simulink model "testmodel2017b"  (R2017b)
settings: Solver=FixedStepDiscrete  StartTime=0.0  StopTime=1000  FixedStep=srate  RelTol=1e-3
PreLoadFcn:
  | model_startup;
model workspace (MAT data in the model file):
  CD_IFBK_GAIN = Simulink.Parameter
  CD_IFBK_GAIN.Value = 0.00279947916667
  CD_IFBK_GAIN.DataType = 'single'
  CD_IFBK_GAIN.Dimensions = [1 1]
  CD_INTEGRATOR_RESET_I = Simulink.Parameter
  CD_INTEGRATOR_RESET_I.Value = 0.01
  CD_INTEGRATOR_RESET_I.DataType = 'single'
  CD_INTEGRATOR_RESET_I.Dimensions = [1 1]
  CD_PRECISION_REF_NOM = Simulink.Parameter
  CD_PRECISION_REF_NOM.Value = 511
  CD_PRECISION_REF_NOM.DataType = 'single'
  CD_PRECISION_REF_NOM.Dimensions = [1 1]
  CD_SOLENOID_RES = Simulink.Parameter
  CD_SOLENOID_RES.Value = 6.1803
  CD_SOLENOID_RES.DataType = 'single'
  CD_SOLENOID_RES.Dimensions = [1 1]
  CD_VBATTERY_GAIN = Simulink.Parameter
  CD_VBATTERY_GAIN.Value = 0.0293360157816
  CD_VBATTERY_GAIN.DataType = 'single'
  CD_VBATTERY_GAIN.Dimensions = [1 1]
  CD_VBATTERY_NOM = Simulink.Parameter
  CD_VBATTERY_NOM.Value = 13.5
  CD_VBATTERY_NOM.DataType = 'single'
  CD_VBATTERY_NOM.Dimensions = [1 1]
  OnPower = Simulink.Signal
  OnPower.DataType = 'boolean'
  OnPower.Dimensions = -1
  OnPower.DimensionsMode = 'auto'
  OnPower.Complexity = 'auto'
  OnPower.SampleTime = -1
  OnPower.SamplingMode = 'auto'
  numOutputs = 6
  srate = 0.001
values from neighbouring files (symbols this model uses):
  CMD_INVERTER_GOTO_OPERATIONAL = Bobcat.Parameter; CreateDefine( CMD_INVERTER_GOTO_OPERATIONAL ,uint8(1) ,'Define' ,'defines.h' )    [enums.m]
  CMD_INVERTER_GOTO_READY = Bobcat.Parameter; CreateDefine( CMD_INVERTER_GOTO_READY       ,uint8(2) ,'Define' ,'defines.h' )    [enums.m]
  CMD_INVERTER_GOTO_STOP = Bobcat.Parameter; CreateDefine( CMD_INVERTER_GOTO_STOP        ,uint8(0) ,'Define' ,'defines.h' )    [enums.m]
  CMD_INVERTER_RUN_FWD = Bobcat.Parameter; CreateDefine( CMD_INVERTER_RUN_FWD          ,uint8(3) ,'Define' ,'defines.h' )    [enums.m]
  INVERTER_CONNECTED = Bobcat.Parameter; CreateDefine( INVERTER_CONNECTED   ,uint8(1) ,'Define' ,'defines.h' )    [enums.m]
  INVERTER_OPERATIONAL = Bobcat.Parameter; CreateDefine( INVERTER_OPERATIONAL ,uint8(2) ,'Define' ,'defines.h' )    [enums.m]
  INVERTER_READY = Bobcat.Parameter; CreateDefine( INVERTER_READY       ,uint8(3) ,'Define' ,'defines.h' )    [enums.m]
  INVERTER_RUN_FWD = Bobcat.Parameter; CreateDefine( INVERTER_RUN_FWD     ,uint8(4) ,'Define' ,'defines.h' )    [enums.m]
  INVERTER_STOP = Bobcat.Parameter; CreateDefine( INVERTER_STOP        ,uint8(0) ,'Define' ,'defines.h' )    [enums.m]
undefined symbols (not defined in the file or in its folder): a, b, c, sigbuilder_block
libraries: simulink x9, hdlsllib x1
CloseFcn:
  | model_end;
settings Model: NumberOfSteps=20000  Creator=cswenson  LastModifiedBy=mmaffeo
settings DataIOCC: SaveOutput=off  SaveTime=off  ReturnWorkspaceOutputs=on
settings OptimizationCC: DefaultParameterBehavior=Inlined  InlineInvariantSignals=on  EnhancedBackFolding=on  PassReuseOutputArgsAs=Individual arguments  StateBitsets=on  DataBitsets=on  LifeSpan=inf  OptimizeBlockOrder=speed  DifferentSizesBufferReuse=on
settings DebuggingCC: ReadBeforeWriteMsg=DisableAll  WriteAfterWriteMsg=DisableAll  WriteAfterReadMsg=DisableAll  AlgebraicLoopMsg=error  ArtificialAlgebraicLoopMsg=error  SaveWithParameterizedLinksMsg=error  BlockPriorityViolationMsg=error  SolverPrmCheckMsg=error  InheritedTsInSrcMsg=error  MultiTaskDSMMsg=none  SigSpecEnsureSampleTimeMsg=error  IntegerOverflowMsg=error  ParameterUnderflowMsg=warning  ParameterTunabilityLossMsg=error  UnderSpecifiedDataTypeMsg=error  UnnecessaryDatatypeConvMsg=warning  VectorMatrixConversionMsg=error  FcnCallInpInsideContextMsg=warning  UnconnectedInputMsg=error  UnconnectedOutputMsg=error  UnconnectedLineMsg=error  SFcnCompatibilityMsg=error  BusObjectLabelMismatch=error  RootOutportRequireBusObject=error  AssertControl=DisableAll  ModelReferenceIOMsg=error  ModelReferenceIOMismatchMessage=error  UnknownTsInhSupMsg=error  ModelReferenceDataLoggingMessage=error  StateNameClashWarn=warning  SFUnexpectedBacktrackingDiag=warning  SFNoUnconditionalDefaultTransitionDiag=warning  SFExecutionAtInitializationDiag=none
settings HardwareCC: ProdBitPerPointer=32  ProdBitPerSizeT=32  ProdBitPerPtrDiffT=32  ProdLargestAtomicInteger=Long  ProdLargestAtomicFloat=Double  ProdWordSize=32  ProdHWDeviceType=ARM Compatible->ARM Cortex  TargetBitPerPointer=64  TargetBitPerSizeT=64  TargetBitPerPtrDiffT=64  TargetLongLongMode=on  TargetIntDivRoundTo=Zero  TargetEndianess=LittleEndian  TargetWordSize=64  TargetHWDeviceType=MATLAB Host
settings ModelReferenceCC: UpdateModelReferenceTargets=IfOutOfDate  PropagateSignalLabelsOutOfModel=off
settings SFSimCC: SimUserSources=SendMsgNow_Blank.cpp  SimUserIncludeDirs=functions  SFSimEcho=off  MATLABDynamicMemAlloc=off
settings SFSimCC: SimCustomHeaderCode=|
  | #include "SendMsgNow.h"
  | #define uint8_t unsigned char
settings RTWCC: SystemTargetFile=bobcat_ert.tlc  GenCodeOnly=on  GenerateMakefile=off  TemplateMakefile=ert_default_tmf  Description=Bobcat Embedded Target derived from RTW-EC  GenerateReport=on  RTWVerbose=off  IncludeHyperlinkInReport=on  LaunchReport=on  PortableWordSizes=on  TargetLang=C++  GenerateTraceInfo=on  GenerateTraceReport=on  GenerateTraceReportSl=on  GenerateTraceReportSf=on  GenerateTraceReportEml=on  GenerateCodeMetricsReport=on  GenerateCodeReplacementReport=on
settings RTWCC: CustomHeaderCode=|
  | #include "cdata.h"
  | #include "ap_can.h"
  | #include "SendMsgNow.h"
  | #include "ap_eeprom.h"
  | #include "ap_bservice_CAN04.h"
settings CodeAppCC: ForceParamTrailComments=on  IgnoreCustomStorageClasses=off  IgnoreTestpoints=on  MangleLength=4  StateflowObjectComments=on  InternalIdentifier=Classic  ReqsInCode=on
settings STFCustomTargetCC: MultiwordLength=256  IncludeMdlTerminateFcn=off  CombineOutputUpdateFcns=on  ERTCustomFileBanners=on  SupportNonFinite=off  SupportComplex=off  SupportNonInlinedSFcns=off  MATLABClassNameForMDSCustomization=Simulink.SoftwareTarget.ERTCustomization  GRTInterface=off  SystemTargetFile=bobcat_ert.tlc
settings ERTTargetCC: ParMdlRefBuildCompliant=off  CompOptLevelCompliant=off  ConcurrentExecutionCompliant=off  IncludeMdlTerminateFcn=off  SupportNonFinite=off  SupportComplex=off  SupportContinuousTime=on  RemoveResetFunc=off  ModelStepFunctionPrototypeControlCompliant=off  CPPClassGenCompliant=off  UseToolchainInfoCompliant=off  InlinedParameterPlacement=NonHierarchical  ERTSrcFileBannerTemplate=bobcat_ert_template.cgt  ERTHdrFileBannerTemplate=bobcat_ert_template.cgt  ERTDataSrcFileTemplate=bobcat_ert_template.cgt  ERTDataHdrFileTemplate=bobcat_ert_template.cgt  ERTCustomFileTemplate=bobcat_file_process.tlc  PreserveExpressionOrder=on  PreserveIfCondition=on  ConvertIfToSwitch=off  SuppressUnreachableDefaultCases=off
settings ConfigComp: CovScope=ReferencedModels  CovIncludeTopModel=off  CovMetricSettings=dw  CovHtmlReporting=on  CovSaveCumulativeToWorkspaceVar=on  CovSaveSingleToWorkspaceVar=on  CovExternalEMLEnable=off  CovSFcnEnable=off

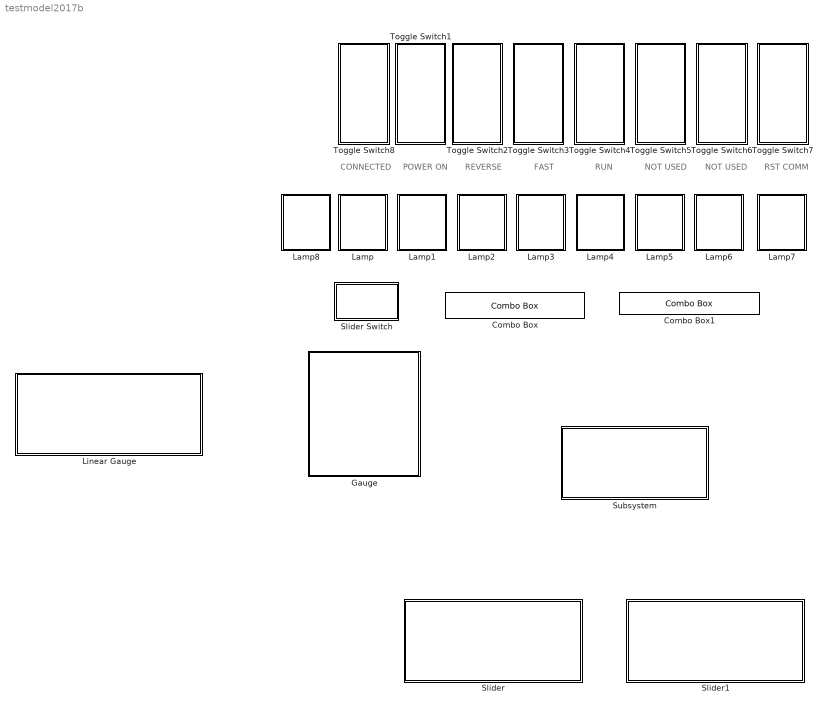
== system testmodel2017b ==
  note: CONNECTED
  note: POWER ON
  note: REVERSE
  note: FAST
  note: RST COMM
  note: RUN
  note: NOT USED
  note: NOT USED
  Combo Box : ComboBox  WebBlockId=8705  ModelName=testmodel2017b  LabelPosition=Top  ShowInitialText=on  SelectedLabel=stop
      settings: Values={{'stop', 'connected', 'operational', 'ready', 'run fwd', 'run rev'}, [0 1 2 3 4 5]}
  Combo Box1 : ComboBox  WebBlockId=8718  ModelName=testmodel2017b  LabelPosition=Hide  ShowInitialText=on  SelectedLabel=Go stop
      settings: Values={{'Go stop', 'Go connected', 'Go operational', 'Go ready', 'Run fwd', 'Run rev'}, [0 1 2 3 4 5]}
  Gauge : Subsystem  DialogController=hmiCreateDDGDialog  IsWebBlock=on  mask(MWDashboardBlock){webBlockId=ca701e44-4673-470a-9dd6-e67335b96dcc, webBlockType=circulargauge, ShowInLibBrowser=on, ShowInitialText=on, HMISrcModelName=testmodel2017b}
      mask prompts: webBlockId "WebBlock Id"; webBlockType "WebBlock Type"; HMISrcModelName "Source Model"
      mask help: SimulinkHMI:dialogs:CircularGaugeDialogDesc
      mask Help: helpview([docroot '/mapfiles/simulink.map'], 'hmi_gauge')
      mask Display:
      | if strcmp(get_param(bdroot(gcb),'BlockDiagramType'), 'library')
      |     image([(matlabroot) '/toolbox/simulink/hmi/icons/CircularGauge.png']);
      | end
  Lamp : Subsystem  DialogController=hmiCreateDDGDialog  IsWebBlock=on  mask(MWDashboardBlock){webBlockId=3d03b230-6085-4f28-82bc-8c8f72340ffd, webBlockType=lamp, ShowInLibBrowser=on, ShowInitialText=on, HMISrcModelName=testmodel2017b}
      mask prompts: webBlockId "WebBlock Id"; webBlockType "WebBlock Type"; HMISrcModelName "Source Model"
      mask help: Display a color that reflects an input value.
      mask Help: helpview([docroot '/mapfiles/simulink.map'], 'hmi_lamp')
      mask Display:
      | if strcmp(get_param(bdroot(gcb),'BlockDiagramType'),'library')
      |  image([(matlabroot) '/toolbox/simulink/hmi/icons/Lamp.png'])
      | end
  Lamp1 : Subsystem  DialogController=hmiCreateDDGDialog  IsWebBlock=on  mask(MWDashboardBlock){webBlockId=3b8bfb2c-1eac-4315-b443-895d23544263, webBlockType=lamp, ShowInLibBrowser=on, ShowInitialText=on, HMISrcModelName=testmodel2017b}
      mask prompts: webBlockId "WebBlock Id"; webBlockType "WebBlock Type"; HMISrcModelName "Source Model"
      mask help: Display a color that reflects an input value.
      mask Help: helpview([docroot '/mapfiles/simulink.map'], 'hmi_lamp')
      mask Display:
      | if strcmp(get_param(bdroot(gcb),'BlockDiagramType'),'library')
      |  image([(matlabroot) '/toolbox/simulink/hmi/icons/Lamp.png'])
      | end
  Lamp2 : Subsystem  DialogController=hmiCreateDDGDialog  IsWebBlock=on  mask(MWDashboardBlock){webBlockId=1077b2a3-7ee6-4687-bbb4-987db73cae4f, webBlockType=lamp, ShowInLibBrowser=on, ShowInitialText=on, HMISrcModelName=testmodel2017b}
      mask prompts: webBlockId "WebBlock Id"; webBlockType "WebBlock Type"; HMISrcModelName "Source Model"
      mask help: Display a color that reflects an input value.
      mask Help: helpview([docroot '/mapfiles/simulink.map'], 'hmi_lamp')
      mask Display:
      | if strcmp(get_param(bdroot(gcb),'BlockDiagramType'),'library')
      |  image([(matlabroot) '/toolbox/simulink/hmi/icons/Lamp.png'])
      | end
  Lamp3 : Subsystem  DialogController=hmiCreateDDGDialog  IsWebBlock=on  mask(MWDashboardBlock){webBlockId=5a2165d5-e830-43a3-9a69-8f3d244f6c12, webBlockType=lamp, ShowInLibBrowser=on, ShowInitialText=on, HMISrcModelName=testmodel2017b}
      mask prompts: webBlockId "WebBlock Id"; webBlockType "WebBlock Type"; HMISrcModelName "Source Model"
      mask help: Display a color that reflects an input value.
      mask Help: helpview([docroot '/mapfiles/simulink.map'], 'hmi_lamp')
      mask Display:
      | if strcmp(get_param(bdroot(gcb),'BlockDiagramType'),'library')
      |  image([(matlabroot) '/toolbox/simulink/hmi/icons/Lamp.png'])
      | end
  Lamp4 : Subsystem  DialogController=hmiCreateDDGDialog  IsWebBlock=on  mask(MWDashboardBlock){webBlockId=2857e801-db19-4a7d-a036-5bbc043663b6, webBlockType=lamp, ShowInLibBrowser=on, ShowInitialText=on, HMISrcModelName=testmodel2017b}
      mask prompts: webBlockId "WebBlock Id"; webBlockType "WebBlock Type"; HMISrcModelName "Source Model"
      mask help: Display a color that reflects an input value.
      mask Help: helpview([docroot '/mapfiles/simulink.map'], 'hmi_lamp')
      mask Display:
      | if strcmp(get_param(bdroot(gcb),'BlockDiagramType'),'library')
      |  image([(matlabroot) '/toolbox/simulink/hmi/icons/Lamp.png'])
      | end
  Lamp5 : Subsystem  DialogController=hmiCreateDDGDialog  IsWebBlock=on  mask(MWDashboardBlock){webBlockId=4482e485-1c61-4683-8091-409276114980, webBlockType=lamp, ShowInLibBrowser=on, ShowInitialText=on, HMISrcModelName=testmodel2017b}
      mask prompts: webBlockId "WebBlock Id"; webBlockType "WebBlock Type"; HMISrcModelName "Source Model"
      mask help: Display a color that reflects an input value.
      mask Help: helpview([docroot '/mapfiles/simulink.map'], 'hmi_lamp')
      mask Display:
      | if strcmp(get_param(bdroot(gcb),'BlockDiagramType'),'library')
      |  image([(matlabroot) '/toolbox/simulink/hmi/icons/Lamp.png'])
      | end
  Lamp6 : Subsystem  DialogController=hmiCreateDDGDialog  IsWebBlock=on  mask(MWDashboardBlock){webBlockId=9855c58a-8830-4368-a696-a0d1540bb0ee, webBlockType=lamp, ShowInLibBrowser=on, ShowInitialText=on, HMISrcModelName=testmodel2017b}
      mask prompts: webBlockId "WebBlock Id"; webBlockType "WebBlock Type"; HMISrcModelName "Source Model"
      mask help: Display a color that reflects an input value.
      mask Help: helpview([docroot '/mapfiles/simulink.map'], 'hmi_lamp')
      mask Display:
      | if strcmp(get_param(bdroot(gcb),'BlockDiagramType'),'library')
      |  image([(matlabroot) '/toolbox/simulink/hmi/icons/Lamp.png'])
      | end
  Lamp7 : Subsystem  DialogController=hmiCreateDDGDialog  IsWebBlock=on  mask(MWDashboardBlock){webBlockId=786d7a47-f623-41eb-b7ff-b095192b59d1, webBlockType=lamp, ShowInLibBrowser=on, ShowInitialText=on, HMISrcModelName=testmodel2017b}
      mask prompts: webBlockId "WebBlock Id"; webBlockType "WebBlock Type"; HMISrcModelName "Source Model"
      mask help: Display a color that reflects an input value.
      mask Help: helpview([docroot '/mapfiles/simulink.map'], 'hmi_lamp')
      mask Display:
      | if strcmp(get_param(bdroot(gcb),'BlockDiagramType'),'library')
      |  image([(matlabroot) '/toolbox/simulink/hmi/icons/Lamp.png'])
      | end
  Lamp8 : Subsystem  DialogController=hmiCreateDDGDialog  IsWebBlock=on  mask(MWDashboardBlock){webBlockId=bc0dacb4-7449-4962-80f3-d142238d4a2f, webBlockType=lamp, ShowInLibBrowser=on, ShowInitialText=on, HMISrcModelName=testmodel2017b}
      mask prompts: webBlockId "WebBlock Id"; webBlockType "WebBlock Type"; HMISrcModelName "Source Model"
      mask help: Display a color that reflects an input value.
      mask Help: helpview([docroot '/mapfiles/simulink.map'], 'hmi_lamp')
      mask Display:
      | if strcmp(get_param(bdroot(gcb),'BlockDiagramType'),'library')
      |  image([(matlabroot) '/toolbox/simulink/hmi/icons/Lamp.png'])
      | end
  Linear Gauge : Subsystem  DialogController=hmiCreateDDGDialog  IsWebBlock=on  mask(MWDashboardBlock){webBlockId=7f63c228-2e19-4776-af30-abd338e55317, webBlockType=lineargauge, ShowInLibBrowser=on, ShowInitialText=on, HMISrcModelName=testmodel2017b}
      mask prompts: webBlockId "WebBlock Id"; webBlockType "WebBlock Type"; HMISrcModelName "Source Model"
      mask help: SimulinkHMI:dialogs:LinearGaugeDialogDesc
      mask Help: helpview([docroot '/mapfiles/simulink.map'], 'hmi_linear_gauge')
      mask Display:
      | if strcmp(get_param(bdroot(gcb),'BlockDiagramType'), 'library')
      |     image([(matlabroot) '/toolbox/simulink/hmi/icons/LinearGauge.png']);
      | end
  Slider : Subsystem  DialogController=hmiCreateDDGDialog  IsWebBlock=on  mask(MWDashboardBlock){webBlockId=fa958995-471b-4ba4-bec5-340cf4a0c4a4, webBlockType=slider, ShowInLibBrowser=on, ShowInitialText=on, HMISrcModelName=testmodel2017b}
      mask prompts: webBlockId "WebBlock Id"; webBlockType "WebBlock Type"; HMISrcModelName "Source Model"
      mask help: SimulinkHMI:dialogs:SliderDialogDesc
      mask Help: helpview([docroot '/mapfiles/simulink.map'], 'hmi_slider')
      mask Display:
      | if strcmp(get_param(bdroot(gcb),'BlockDiagramType'), 'library')
      |     image([(matlabroot) '/toolbox/simulink/hmi/icons/Slider.png']);
      | end
  Slider Switch : Subsystem  DialogController=hmiCreateDDGDialog  IsWebBlock=on  mask(MWDashboardBlock){webBlockId=e8f953b1-b3fd-4705-a0b6-97bfe8724c95, webBlockType=sliderswitch, ShowInLibBrowser=on, ShowInitialText=on, HMISrcModelName=testmodel2017b}
      mask prompts: webBlockId "WebBlock Id"; webBlockType "WebBlock Type"; HMISrcModelName "Source Model"
      mask help: Set on/off value to tune parameters or variables.
      mask Help: helpview([docroot '/mapfiles/simulink.map'], 'hmi_switch')
      mask Display:
      | if strcmp(get_param(bdroot(gcb),'BlockDiagramType'),'library')
      |  image([(matlabroot) '/toolbox/simulink/hmi/icons/SliderSwitch.png'])
      | end
  Slider1 : Subsystem  DialogController=hmiCreateDDGDialog  IsWebBlock=on  mask(MWDashboardBlock){webBlockId=517096a1-4060-40ba-819b-9a3d476b2f75, webBlockType=slider, ShowInLibBrowser=on, ShowInitialText=on, HMISrcModelName=testmodel2017b}
      mask prompts: webBlockId "WebBlock Id"; webBlockType "WebBlock Type"; HMISrcModelName "Source Model"
      mask help: SimulinkHMI:dialogs:SliderDialogDesc
      mask Help: helpview([docroot '/mapfiles/simulink.map'], 'hmi_slider')
      mask Display:
      | if strcmp(get_param(bdroot(gcb),'BlockDiagramType'), 'library')
      |     image([(matlabroot) '/toolbox/simulink/hmi/icons/Slider.png']);
      | end
  Subsystem : Subsystem
  Toggle Switch1 : Subsystem  DialogController=hmiCreateDDGDialog  IsWebBlock=on  mask(MWDashboardBlock){webBlockId=47589691-0491-44e5-b52c-3802481a810c, webBlockType=toggleswitch, ShowInLibBrowser=on, ShowInitialText=on, HMISrcModelName=testmodel2017b}
      mask prompts: webBlockId "WebBlock Id"; webBlockType "WebBlock Type"; HMISrcModelName "Source Model"
      mask help: SimulinkHMI:dialogs:SwitchDialogDesc
      mask Help: helpview([docroot '/mapfiles/simulink.map'], 'hmi_toggle_switch')
      mask Display:
      | if strcmp(get_param(bdroot(gcb),'BlockDiagramType'), 'library')
      |     image([(matlabroot) '/toolbox/simulink/hmi/icons/ToggleSwitch.png']);
      | end
  Toggle Switch2 : Subsystem  DialogController=hmiCreateDDGDialog  IsWebBlock=on  mask(MWDashboardBlock){webBlockId=03349644-d7f0-4194-b582-00e40be6aa1b, webBlockType=toggleswitch, ShowInLibBrowser=on, ShowInitialText=on, HMISrcModelName=testmodel2017b}
      mask prompts: webBlockId "WebBlock Id"; webBlockType "WebBlock Type"; HMISrcModelName "Source Model"
      mask help: SimulinkHMI:dialogs:SwitchDialogDesc
      mask Help: helpview([docroot '/mapfiles/simulink.map'], 'hmi_toggle_switch')
      mask Display:
      | if strcmp(get_param(bdroot(gcb),'BlockDiagramType'), 'library')
      |     image([(matlabroot) '/toolbox/simulink/hmi/icons/ToggleSwitch.png']);
      | end
  Toggle Switch3 : Subsystem  DialogController=hmiCreateDDGDialog  IsWebBlock=on  mask(MWDashboardBlock){webBlockId=8be4c630-fc00-43e9-b3e7-282d6444acbb, webBlockType=toggleswitch, ShowInLibBrowser=on, ShowInitialText=on, HMISrcModelName=testmodel2017b}
      mask prompts: webBlockId "WebBlock Id"; webBlockType "WebBlock Type"; HMISrcModelName "Source Model"
      mask help: SimulinkHMI:dialogs:SwitchDialogDesc
      mask Help: helpview([docroot '/mapfiles/simulink.map'], 'hmi_toggle_switch')
      mask Display:
      | if strcmp(get_param(bdroot(gcb),'BlockDiagramType'), 'library')
      |     image([(matlabroot) '/toolbox/simulink/hmi/icons/ToggleSwitch.png']);
      | end
  Toggle Switch4 : Subsystem  DialogController=hmiCreateDDGDialog  IsWebBlock=on  mask(MWDashboardBlock){webBlockId=669c9247-3514-4664-88b6-ae32ca600e88, webBlockType=toggleswitch, ShowInLibBrowser=on, ShowInitialText=on, HMISrcModelName=testmodel2017b}
      mask prompts: webBlockId "WebBlock Id"; webBlockType "WebBlock Type"; HMISrcModelName "Source Model"
      mask help: SimulinkHMI:dialogs:SwitchDialogDesc
      mask Help: helpview([docroot '/mapfiles/simulink.map'], 'hmi_toggle_switch')
      mask Display:
      | if strcmp(get_param(bdroot(gcb),'BlockDiagramType'), 'library')
      |     image([(matlabroot) '/toolbox/simulink/hmi/icons/ToggleSwitch.png']);
      | end
  Toggle Switch5 : Subsystem  DialogController=hmiCreateDDGDialog  IsWebBlock=on  mask(MWDashboardBlock){webBlockId=9df9911a-db6a-4f88-9175-2bee3af0034b, webBlockType=toggleswitch, ShowInLibBrowser=on, ShowInitialText=on, HMISrcModelName=testmodel2017b}
      mask prompts: webBlockId "WebBlock Id"; webBlockType "WebBlock Type"; HMISrcModelName "Source Model"
      mask help: SimulinkHMI:dialogs:SwitchDialogDesc
      mask Help: helpview([docroot '/mapfiles/simulink.map'], 'hmi_toggle_switch')
      mask Display:
      | if strcmp(get_param(bdroot(gcb),'BlockDiagramType'), 'library')
      |     image([(matlabroot) '/toolbox/simulink/hmi/icons/ToggleSwitch.png']);
      | end
  Toggle Switch6 : Subsystem  DialogController=hmiCreateDDGDialog  IsWebBlock=on  mask(MWDashboardBlock){webBlockId=26248c20-b423-42ea-b6b6-d3060b4fe5f6, webBlockType=toggleswitch, ShowInLibBrowser=on, ShowInitialText=on, HMISrcModelName=testmodel2017b}
      mask prompts: webBlockId "WebBlock Id"; webBlockType "WebBlock Type"; HMISrcModelName "Source Model"
      mask help: SimulinkHMI:dialogs:SwitchDialogDesc
      mask Help: helpview([docroot '/mapfiles/simulink.map'], 'hmi_toggle_switch')
      mask Display:
      | if strcmp(get_param(bdroot(gcb),'BlockDiagramType'), 'library')
      |     image([(matlabroot) '/toolbox/simulink/hmi/icons/ToggleSwitch.png']);
      | end
  Toggle Switch7 : Subsystem  DialogController=hmiCreateDDGDialog  IsWebBlock=on  mask(MWDashboardBlock){webBlockId=519b3b3b-eed3-4fa3-8c24-ef273513dd86, webBlockType=toggleswitch, ShowInLibBrowser=on, ShowInitialText=on, HMISrcModelName=testmodel2017b}
      mask prompts: webBlockId "WebBlock Id"; webBlockType "WebBlock Type"; HMISrcModelName "Source Model"
      mask help: SimulinkHMI:dialogs:SwitchDialogDesc
      mask Help: helpview([docroot '/mapfiles/simulink.map'], 'hmi_toggle_switch')
      mask Display:
      | if strcmp(get_param(bdroot(gcb),'BlockDiagramType'), 'library')
      |     image([(matlabroot) '/toolbox/simulink/hmi/icons/ToggleSwitch.png']);
      | end
  Toggle Switch8 : Subsystem  DialogController=hmiCreateDDGDialog  IsWebBlock=on  mask(MWDashboardBlock){webBlockId=17c79f1b-60e0-4136-926c-46730ae39f4c, webBlockType=toggleswitch, ShowInLibBrowser=on, ShowInitialText=on, HMISrcModelName=testmodel2017b}
      mask prompts: webBlockId "WebBlock Id"; webBlockType "WebBlock Type"; HMISrcModelName "Source Model"
      mask help: SimulinkHMI:dialogs:SwitchDialogDesc
      mask Help: helpview([docroot '/mapfiles/simulink.map'], 'hmi_toggle_switch')
      mask Display:
      | if strcmp(get_param(bdroot(gcb),'BlockDiagramType'), 'library')
      |     image([(matlabroot) '/toolbox/simulink/hmi/icons/ToggleSwitch.png']);
      | end

== system testmodel2017b/Gauge ==

== system testmodel2017b/Lamp ==

== system testmodel2017b/Lamp1 ==

== system testmodel2017b/Lamp2 ==

== system testmodel2017b/Lamp3 ==

== system testmodel2017b/Lamp4 ==

== system testmodel2017b/Lamp5 ==

== system testmodel2017b/Lamp6 ==

== system testmodel2017b/Lamp7 ==

== system testmodel2017b/Lamp8 ==

== system testmodel2017b/Linear Gauge ==

== system testmodel2017b/Slider ==

== system testmodel2017b/Slider Switch ==

== system testmodel2017b/Slider1 ==

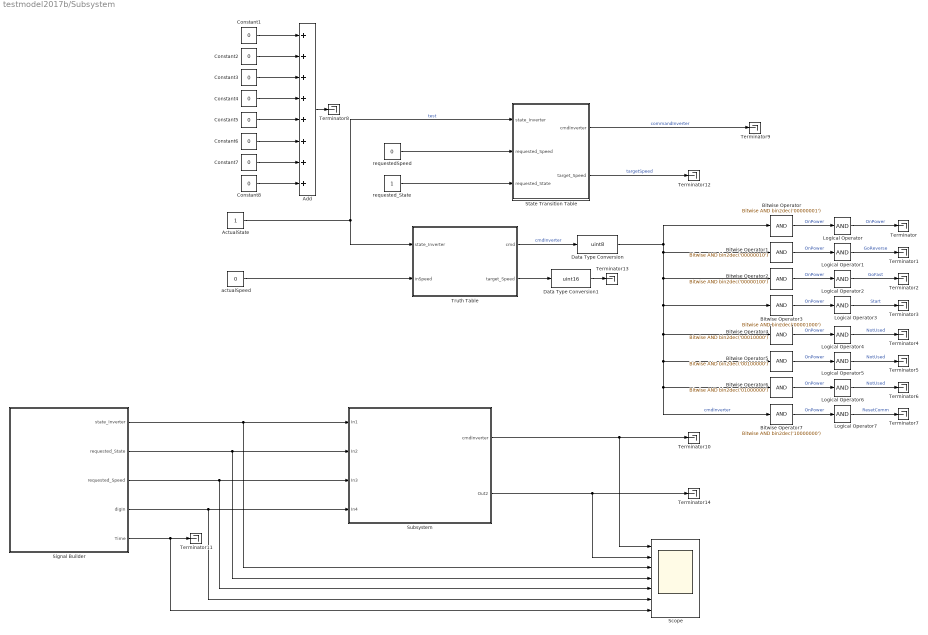
== system testmodel2017b/Subsystem ==
  ActualState : Constant  OutDataTypeStr=uint8
  Add : Sum  Inputs=++++++++  OutDataTypeStr=uint8
  Bitwise Operator : simulink/Logic and Bit Operations/Bitwise Operator  logicop=AND  UseBitMask=on  BitMask=bin2dec('00000001')  BitMaskRealWorld=Stored Integer
  Bitwise Operator1 : simulink/Logic and Bit Operations/Bitwise Operator  logicop=AND  UseBitMask=on  BitMask=bin2dec('00000010')  BitMaskRealWorld=Stored Integer
  Bitwise Operator2 : simulink/Logic and Bit Operations/Bitwise Operator  logicop=AND  UseBitMask=on  BitMask=bin2dec('00000100')  BitMaskRealWorld=Stored Integer
  Bitwise Operator3 : simulink/Logic and Bit Operations/Bitwise Operator  logicop=AND  UseBitMask=on  BitMask=bin2dec('00001000')  BitMaskRealWorld=Stored Integer
  Bitwise Operator4 : simulink/Logic and Bit Operations/Bitwise Operator  logicop=AND  UseBitMask=on  BitMask=bin2dec('00010000')  BitMaskRealWorld=Stored Integer
  Bitwise Operator5 : simulink/Logic and Bit Operations/Bitwise Operator  logicop=AND  UseBitMask=on  BitMask=bin2dec('00100000')  BitMaskRealWorld=Stored Integer
  Bitwise Operator6 : simulink/Logic and Bit Operations/Bitwise Operator  logicop=AND  UseBitMask=on  BitMask=bin2dec('01000000')  BitMaskRealWorld=Stored Integer
  Bitwise Operator7 : simulink/Logic and Bit Operations/Bitwise Operator  logicop=AND  UseBitMask=on  BitMask=bin2dec('10000000')  BitMaskRealWorld=Stored Integer
  Constant{1..8} (8 alike) : Constant  Value=0
  Data Type Conversion : DataTypeConversion  OutDataTypeStr=uint8
  Data Type Conversion1 : DataTypeConversion  OutDataTypeStr=uint16
  Logical Operator{,1..7} (8 alike) : Logic  Inputs=1  AllPortsSameDT=off  OutDataTypeStr=boolean
  Scope : Scope  NumInputPorts=7
  Signal Builder : Subsystem  Tag=STV Subsys  LoadFcn=sigbuilder_block('load',[-1536 0 1536 808.8 ]);  StartFcn=sigbuilder_block('start');  StopFcn=sigbuilder_block('stop');  ClipboardFcn=sigbuilder_block('clipboard');  mask(Sigbuilder block){tuvar=[0:10]}
      mask help: Simulink:masks:SigbuilderBlock_MD
      mask init:
      | if ~strcmp(get_param(bdroot(gcbh),'SimulationStatus'),'stopped') tuvar = sigbuilder_block('maskInit'); end
      settings: CopyFcn=sigbuilder_block('copy');  DeleteFcn=sigbuilder_block('delete');  ModelCloseFcn=sigbuilder_block('modelClose');  PreSaveFcn=sigbuilder_block('preSave');  PauseFcn=sigbuilder_block('pause');  ContinueFcn=sigbuilder_block('continue');  NameChangeFcn=sigbuilder_block('namechange');  OpenFcn=sigbuilder_block('open',[437.6 199.2 550.4 400 ]);  CloseFcn=sigbuilder_block('close');
      mask Display: plot(0, 0, 100, 100,[2, 2, 32, 32, 2], [68, 8, 8, 68, 68],[32, 2], [38, 38], [32, 19, 2],[53, 60, 44], [32, 17, 17, 2],[16, 16, 31, 31]);txt = getActiveGroup(gcbh);text(2, 100, txt,'verticalAlignment', 'top');
  State Transition Table : State Transition Table  TreatAsAtomicUnit=on
  Subsystem : Subsystem
  Terminator{,1..14} (15 alike) : Terminator
  Truth Table : Truth Table  TreatAsAtomicUnit=on
  actualSpeed : Constant  Value=0  OutDataTypeStr=uint16
  requestedSpeed : Constant  Value=0  OutDataTypeStr=uint16
  requested_State : Constant  OutDataTypeStr=uint8
  wires:
  ActualState/1 -> Truth Table/1(state_Inverter), State Transition Table/1(state_Inverter)  "test"
  Constant1/1 -> Add/1
  Constant7/1 -> Add/7
  Constant5/1 -> Add/5
  Constant6/1 -> Add/6
  Constant8/1 -> Add/8
  Constant4/1 -> Add/4
  Constant2/1 -> Add/2
  Constant3/1 -> Add/3
  Logical Operator/1 -> Terminator/1  "OnPower"
  Logical Operator1/1 -> Terminator1/1  "GoReverse"
  Logical Operator4/1 -> Terminator4/1  "NotUsed"
  Logical Operator5/1 -> Terminator5/1  "NotUsed"
  Logical Operator6/1 -> Terminator6/1  "NotUsed"
  Logical Operator7/1 -> Terminator7/1  "ResetComm"
  Data Type Conversion/1 -> Bitwise Operator7/1, Bitwise Operator6/1, Bitwise Operator5/1, Bitwise Operator4/1, Bitwise Operator3/1, Bitwise Operator2/1, Bitwise Operator1/1, Bitwise Operator/1  "cmdInverter"
  Bitwise Operator/1 -> Logical Operator/1  "OnPower"
  Bitwise Operator1/1 -> Logical Operator1/1  "OnPower"
  Bitwise Operator2/1 -> Logical Operator2/1  "OnPower"
  Bitwise Operator3/1 -> Logical Operator3/1  "OnPower"
  Logical Operator2/1 -> Terminator2/1  "GoFast"
  Logical Operator3/1 -> Terminator3/1  "Start"
  Bitwise Operator7/1 -> Logical Operator7/1  "OnPower"
  Bitwise Operator4/1 -> Logical Operator4/1  "OnPower"
  Bitwise Operator6/1 -> Logical Operator6/1  "OnPower"
  Bitwise Operator5/1 -> Logical Operator5/1  "OnPower"
  Add/1 -> Terminator8/1
  actualSpeed/1 -> Truth Table/2(inSpeed)
  Truth Table/1(cmd) -> Data Type Conversion/1  "cmdInverter"
  Truth Table/2(target_Speed) -> Data Type Conversion1/1
  requested_State/1 -> State Transition Table/3(requested_State)
  State Transition Table/1(cmdInverter) -> Terminator9/1  "commandInverter"
  requestedSpeed/1 -> State Transition Table/2(requested_Speed)
  Signal Builder/2(requested_State) -> Subsystem/2(In2), Scope/4
  Signal Builder/3(requested_Speed) -> Subsystem/3(In3), Scope/5
  Signal Builder/1(state_Inverter) -> Subsystem/1(In1), Scope/3
  Signal Builder/5(Time) -> Scope/7, Terminator11/1
  State Transition Table/2(target_Speed) -> Terminator12/1  "targetSpeed"
  Data Type Conversion1/1 -> Terminator13/1
  Signal Builder/4(digIn) -> Subsystem/4(In4), Scope/6
  Subsystem/2(Out2) -> Terminator14/1, Scope/2
  Subsystem/1(cmdInverter) -> Terminator10/1, Scope/1

== system testmodel2017b/Toggle Switch1 ==

== system testmodel2017b/Toggle Switch2 ==

== system testmodel2017b/Toggle Switch3 ==

== system testmodel2017b/Toggle Switch4 ==

== system testmodel2017b/Toggle Switch5 ==

== system testmodel2017b/Toggle Switch6 ==

== system testmodel2017b/Toggle Switch7 ==

== system testmodel2017b/Toggle Switch8 ==

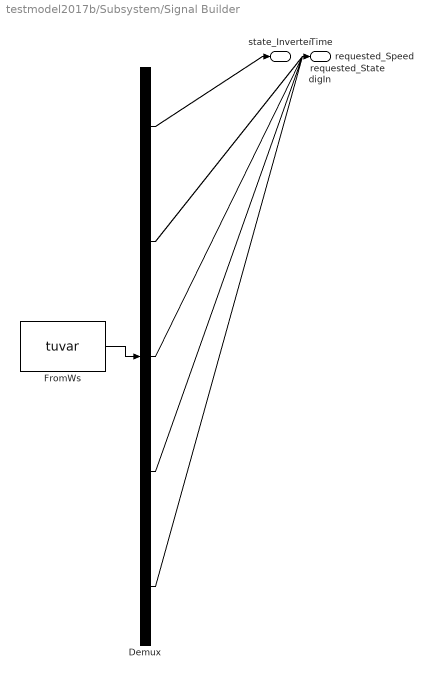
== system testmodel2017b/Subsystem/Signal Builder ==
  Demux : Demux  Tag=STV Demux  Outputs=5
  FromWs : FromWorkspace  Tag=STV FromWs  VariableName=tuvar  SampleTime=0
      SigBuilderData=|
      | common.afterFinalStr = 'Extrapolate'
      | common.sampleTime = 0
      | dataSet(1).timeRange = [0 1000]
      | dataSet(1).name = 'Normal Sequence'
      | dataSet(2).timeRange = [0 1000]
      | dataSet(2).name = 'EmergenzyStop'
      | dataSet(3).timeRange = [0 1000]
      | dataSet(3).name = 'SeatBar'
      | sbobj.Name = 'Signal Builder'
      | sbobj.Groups(1).Name = 'Normal Sequence'
      | sbobj.Groups(1).Signals(1).Name = 'state_Inverter'
      | sbobj.Groups(1).Signals(1).XData = [0 10 20 30 40 50 60 70 80 90 100 110 120 130 140 150 160 170 180 190 200 210 220 230 240 250 260 270 280 290 300 310 320 330 340 350 360 370 380 390 400 410 420 430 440 450 460 470 480 490 500 510 520 530 540 550 560 570 580 590 600 610 620 630 640 650 660 670 680 690 700 710 720 730 740 750 760 770 780 790 800 810 820 830 840 850 860 870 880 890 900 910 920 930 940 950 960 970 980 990 1000]
      | sbobj.Groups(1).Signals(1).YData = [0 0 0 0 0 0 0 0 0 0 0 1 1 1 1 1 1 1 1 1 1 1 1 1 2 2 2 2 2 2 2 2 2 2 2 3 3 3 3 3 3 3 3 3 3 3 3 4 4 4 4 4 4 4 4 4 4 5 5 5 5 5 5 5 5 6 6 6 6 6 6 6 6 6 6 6 6 6 6 6 6 6 6 6 6 6 6 6 6 6 6 6 6 6 6 6 6 6 6 6 6]
      | sbobj.Groups(1).Signals(2).Name = 'requested_State'
      | sbobj.Groups(1).Signals(2).XData = [0 10 20 30 40 50 60 70 80 90 100 110 120 130 140 150 160 170 180 190 200 210 220 230 240 250 260 270 280 290 300 310 320 330 340 350 360 370 380 390 400 410 420 430 440 450 460 470 480 490 500 510 520 530 540 550 560 570 580 590 600 610 620 630 640 650 660 670 680 690 700 710 720 730 740 750 760 770 780 790 800 810 820 830 840 850 860 870 880 890 900 910 920 930 940 950 960 970 980 990 1000]
      | sbobj.Groups(1).Signals(2).YData = [0 0 0 0 0 1 1 1 1 1 1 1 1 1 1 1 1 1 2 2 2 2 2 2 2 2 2 2 2 3 3 3 3 3 3 3 3 3 3 3 3 4 4 4 4 4 4 4 4 4 4 5 5 5 5 5 5 5 5 6 6 6 6 6 6 6 6 6 6 6 6 6 6 6 6 6 6 6 6 6 6 6 6 6 6 6 6 6 6 6 6 6 6 6 6 6 6 6 6 6 6]
      | sbobj.Groups(1).Signals(3).Name = 'requested_Speed'
      | sbobj.Groups(1).Signals(3).XData = [0 10 20 30 40 50 60 70 80 90 100 110 120 130 140 150 160 170 180 190 200 210 220 230 240 250 260 270 280 290 300 310 320 330 340 350 360 370 380 390 400 410 420 430 440 450 460 470 480 490 500 510 520 530 540 550 560 570 580 590 600 610 620 630 640 650 660 670 680 690 700 710 720 730 740 750 760 770 780 790 800 810 820 830 840 850 860 870 880 890 900 910 920 930 940 950 960 970 980 990 1000]
      | sbobj.Groups(1).Signals(3).YData = [0 0 0 0 0 0 0 0 0 0 0 0 0 0 0 0 0 0 0 0 0 0 0 0 0 0 0 0 0 0 0 0 0 0 0 0 0 0 0 0 0 0 0 0 0 0 0 0 0 0 0 0 0 0 0 0 0 0 0 25 50 75 100 125 150 175 200 225 250 275 300 325 350 375 400 425 450 475 500 525 550 575 600 625 650 675 700 725 750 775 800 825 850 875 900 925 950 975 1000 1025 1050]
      | sbobj.Groups(1).Signals(4).Name = 'digIn'
      | sbobj.Groups(1).Signals(4).XData = [0 10 20 30 40 50 60 70 80 90 100 110 120 130 140 150 160 170 180 190 200 210 220 230 240 250 260 270 280 290 300 310 320 330 340 350 360 370 380 390 400 410 420 430 440 450 460 470 480 490 500 510 520 530 540 550 560 570 580 590 600 610 620 630 640 650 660 670 680 690 700 710 720 730 740 750 760 770 780 790 800 810 820 830 840 850 860 870 880 890 900 910 920 930 940 950 960 970 980 990 1000]
      | sbobj.Groups(1).Signals(4).YData = [0 1 1 1 1 1 1 1 1 1 1 1 1 1 1 1 1 1 1 1 1 1 1 1 1 1 1 1 1 1 1 1 1 1 1 1 1 1 1 1 1 1 1 1 1 1 1 1 1 1 1 1 1 1 1 1 1 1 1 1 1 1 1 1 1 1 1 1 1 1 1 1 1 1 1 1 1 1 1 1 1 1 1 1 1 1 1 1 1 1 1 1 1 1 1 1 1 1 1 1 1]
      | sbobj.Groups(1).Signals(5).Name = 'Time'
      | sbobj.Groups(1).Signals(5).XData = [0 10 20 30 40 50 60 70 80 90 100 110 120 130 140 150 160 170 180 190 200 210 220 230 240 250 260 270 280 290 300 310 320 330 340 350 360 370 380 390 400 410 420 430 440 450 460 470 480 490 500 510 520 530 540 550 560 570 580 590 600 610 620 630 640 650 660 670 680 690 700 710 720 730 740 750 760 770 780 790 800 810 820 830 840 850 860 870 880 890 900 910 920 930 940 950 960 970 980 990 1000]
      | sbobj.Groups(1).Signals(5).YData = [0 10 20 30 40 50 60 70 80 90 100 110 120 130 140 150 160 170 180 190 200 210 220 230 240 250 260 270 280 290 300 310 320 330 340 350 360 370 380 390 400 410 420 430 440 450 460 470 480 490 500 510 520 530 540 550 560 570 580 590 600 610 620 630 640 650 660 670 680 690 700 710 720 730 740 750 760 770 780 790 800 810 820 830 840 850 860 870 880 890 900 910 920 930 940 950 960 970 980 990 1000]
      | sbobj.Groups(1).TimeRange = [0 1000]
      | sbobj.Groups(2).Name = 'EmergenzyStop'
      | sbobj.Groups(2).Signals(1).Name = 'state_Inverter'
      | sbobj.Groups(2).Signals(1).XData = [0 10 20 30 40 50 60 70 80 90 100 110 120 130 140 150 160 170 180 190 200 210 220 230 240 250 260 270 280 290 300 310 320 330 340 350 360 370 380 390 400 410 420 430 440 450 460 470 480 490 500 510 520 530 540 550 560 570 580 590 600 610 620 630 640 650 660 670 680 690 700 710 720 730 740 750 760 770 780 790 800 810 820 830 840 850 860 870 880 890 900 910 920 930 940 950 960 970 980 990 1000]
      | sbobj.Groups(2).Signals(1).YData = [0 0 0 1 1 2 2 3 3 4 4 5 5 6 6 0 0 0 0 0 0 0 0 0 0 0 0 0 0 0 0 0 0 0 0 0 0 0 0 0 0 0 0 0 0 0 0 0 0 0 0 0 0 0 0 0 0 0 0 0 0 0 0 0 0 0 0 0 0 0 0 0 0 0 0 0 0 0 0 0 0 0 0 0 0 0 0 0 0 0 0 0 0 0 0 0 0 0 0 0 0]
      | sbobj.Groups(2).Signals(2).Name = 'requested_State'
      | sbobj.Groups(2).Signals(2).XData = [0 10 20 30 40 50 60 70 80 90 100 110 120 130 140 150 160 170 180 190 200 210 220 230 240 250 260 270 280 290 300 310 320 330 340 350 360 370 380 390 400 410 420 430 440 450 460 470 480 490 500 510 520 530 540 550 560 570 580 590 600 610 620 630 640 650 660 670 680 690 700 710 720 730 740 750 760 770 780 790 800 810 820 830 840 850 860 870 880 890 900 910 920 930 940 950 960 970 980 990 1000]
      | sbobj.Groups(2).Signals(2).YData = [0 0 1 1 2 2 3 3 4 4 5 5 6 6 6 6 6 6 6 6 6 6 0 0 0 0 0 0 0 0 0 0 0 0 0 0 0 0 0 0 0 0 0 0 0 0 0 0 0 0 0 0 0 0 0 0 0 0 0 0 0 0 0 0 0 0 0 0 0 0 0 0 0 0 0 0 0 0 0 0 0 0 0 0 0 0 0 0 0 0 0 0 0 0 0 0 0 0 0 0 0]
      | sbobj.Groups(2).Signals(3).Name = 'requested_Speed'
      | sbobj.Groups(2).Signals(3).XData = [0 10 20 30 40 50 60 70 80 90 100 110 120 130 140 150 160 170 180 190 200 210 220 230 240 250 260 270 280 290 300 310 320 330 340 350 360 370 380 390 400 410 420 430 440 450 460 470 480 490 500 510 520 530 540 550 560 570 580 590 600 610 620 630 640 650 660 670 680 690 700 710 720 730 740 750 760 770 780 790 800 810 820 830 840 850 860 870 880 890 900 910 920 930 940 950 960 970 980 990 1000]
      | sbobj.Groups(2).Signals(3).YData = [1500 1500 1500 1500 1500 1500 1500 1500 1500 1500 1500 1500 1500 1500 1500 1500 1500 1500 1500 1500 1500 1500 1500 1500 1500 1500 1500 1500 1500 1500 1500 1500 1500 1500 1500 1500 1500 1500 1500 1500 1500 1500 1500 1500 1500 1500 1500 1500 1500 1500 1500 1500 1500 1500 1500 1500 1500 1500 1500 1500 1500 1500 1500 1500 1500 1500 1500 1500 1500 1500 1500 1500 1500 1500 1500 1500 1500 1500 1500 1500 1500 1500 1500 1500 1500 1500 1500 1500 1500 1500 1500 1500 1500 1500 1500 1500 1500 1500 1500 1500 1500]
      | sbobj.Groups(2).Signals(4).Name = 'digIn'
      | sbobj.Groups(2).Signals(4).XData = [0 10 20 30 40 50 60 70 80 90 100 110 120 130 140 150 160 170 180 190 200 210 220 230 240 250 260 270 280 290 300 310 320 330 340 350 360 370 380 390 400 410 420 430 440 450 460 470 480 490 500 510 520 530 540 550 560 570 580 590 600 610 620 630 640 650 660 670 680 690 700 710 720 730 740 750 760 770 780 790 800 810 820 830 840 850 860 870 880 890 900 910 920 930 940 950 960 970 980 990 1000]
      | sbobj.Groups(2).Signals(4).YData = [0 1 1 1 1 1 1 1 1 1 1 1 1 1 1 1 1 1 1 1 1 1 1 1 1 1 1 1 1 1 1 1 1 1 1 1 1 1 1 1 1 1 1 1 1 1 1 1 1 1 1 1 1 1 1 1 1 1 1 1 1 1 1 1 1 1 1 1 1 1 1 1 1 1 1 1 1 1 1 1 1 1 1 1 1 1 1 1 1 1 1 1 1 1 1 1 1 1 1 1 1]
      | sbobj.Groups(2).Signals(5).Name = 'Time'
      | sbobj.Groups(2).Signals(5).XData = [0 10 20 30 40 50 60 70 80 90 100 110 120 130 140 150 160 170 180 190 200 210 220 230 240 250 260 270 280 290 300 310 320 330 340 350 360 370 380 390 400 410 420 430 440 450 460 470 480 490 500 510 520 530 540 550 560 570 580 590 600 610 620 630 640 650 660 670 680 690 700 710 720 730 740 750 760 770 780 790 800 810 820 830 840 850 860 870 880 890 900 910 920 930 940 950 960 970 980 990 1000]
      | sbobj.Groups(2).Signals(5).YData = [0 10 20 30 40 50 60 70 80 90 100 110 120 130 140 150 160 170 180 190 200 210 220 230 240 250 260 270 280 290 300 310 320 330 340 350 360 370 380 390 400 410 420 430 440 450 460 470 480 490 500 510 520 530 540 550 560 570 580 590 600 610 620 630 640 650 660 670 680 690 700 710 720 730 740 750 760 770 780 790 800 810 820 830 840 850 860 870 880 890 900 910 920 930 940 950 960 970 980 990 1000]
      | sbobj.Groups(2).TimeRange = [0 1000]
      | sbobj.Groups(3).Name = 'SeatBar'
      | sbobj.Groups(3).Signals(1).Name = 'state_Inverter'
      | sbobj.Groups(3).Signals(1).XData = [0 10 20 30 40 50 60 70 80 90 100 110 120 130 140 150 160 170 180 190 200 210 220 230 240 250 260 270 280 290 300 310 320 330 340 350 360 370 380 390 400 410 420 430 440 450 460 470 480 490 500 510 520 530 540 550 560 570 580 590 600 610 620 630 640 650 660 670 680 690 700 710 720 730 740 750 760 770 780 790 800 810 820 830 840 850 860 870 880 890 900 910 920 930 940 950 960 970 980 990 1000]
      | sbobj.Groups(3).Signals(1).YData = [0 0 0 1 1 2 2 3 3 4 4 5 5 6 6 0 0 0 0 0 0 0 0 0 0 0 0 0 0 0 0 0 0 0 0 0 0 0 0 0 0 0 0 0 0 0 0 0 0 0 0 0 0 0 0 0 0 0 0 0 0 0 0 0 0 0 0 0 0 0 0 0 0 0 0 0 0 0 0 0 0 0 0 0 0 0 0 0 0 0 0 0 0 0 0 0 0 0 0 0 0]
      | sbobj.Groups(3).Signals(2).Name = 'requested_State'
      | sbobj.Groups(3).Signals(2).XData = [0 10 20 30 40 50 60 70 80 90 100 110 120 130 140 150 160 170 180 190 200 210 220 230 240 250 260 270 280 290 300 310 320 330 340 350 360 370 380 390 400 410 420 430 440 450 460 470 480 490 500 510 520 530 540 550 560 570 580 590 600 610 620 630 640 650 660 670 680 690 700 710 720 730 740 750 760 770 780 790 800 810 820 830 840 850 860 870 880 890 900 910 920 930 940 950 960 970 980 990 1000]
      | sbobj.Groups(3).Signals(2).YData = [0 0 1 1 2 2 3 3 4 4 5 5 6 6 6 6 6 6 6 6 6 6 0 0 0 0 0 0 0 0 0 0 0 0 0 0 0 0 0 0 0 0 0 0 0 0 0 0 0 0 0 0 0 0 0 0 0 0 0 0 0 0 0 0 0 0 0 0 0 0 0 0 0 0 0 0 0 0 0 0 0 0 0 0 0 0 0 0 0 0 0 0 0 0 0 0 0 0 0 0 0]
      | sbobj.Groups(3).Signals(3).Name = 'requested_Speed'
      | sbobj.Groups(3).Signals(3).XData = [0 10 20 30 40 50 60 70 80 90 100 110 120 130 140 150 160 170 180 190 200 210 220 230 240 250 260 270 280 290 300 310 320 330 340 350 360 370 380 390 400 410 420 430 440 450 460 470 480 490 500 510 520 530 540 550 560 570 580 590 600 610 620 630 640 650 660 670 680 690 700 710 720 730 740 750 760 770 780 790 800 810 820 830 840 850 860 870 880 890 900 910 920 930 940 950 960 970 980 990 1000]
      | sbobj.Groups(3).Signals(3).YData = [1500 1500 1500 1500 1500 1500 1500 1500 1500 1500 1500 1500 1500 1500 1500 1500 1500 1500 1500 1500 1500 1500 1500 1500 1500 1500 1500 1500 1500 1500 1500 1500 1500 1500 1500 1500 1500 1500 1500 1500 1500 1500 1500 1500 1500 1500 1500 1500 1500 1500 1500 1500 1500 1500 1500 1500 1500 1500 1500 1500 1500 1500 1500 1500 1500 1500 1500 1500 1500 1500 1500 1500 1500 1500 1500 1500 1500 1500 1500 1500 1500 1500 1500 1500 1500 1500 1500 1500 1500 1500 1500 1500 1500 1500 1500 1500 1500 1500 1500 1500 1500]
      | sbobj.Groups(3).Signals(4).Name = 'digIn'
      | sbobj.Groups(3).Signals(4).XData = [0 10 20 30 40 50 60 70 80 90 100 110 120 130 140 150 160 170 180 190 200 210 220 230 240 250 260 270 280 290 300 310 320 330 340 350 360 370 380 390 400 410 420 430 440 450 460 470 480 490 500 510 520 530 540 550 560 570 580 590 600 610 620 630 640 650 660 670 680 690 700 710 720 730 740 750 760 770 780 790 800 810 820 830 840 850 860 870 880 890 900 910 920 930 940 950 960 970 980 990 1000]
      | sbobj.Groups(3).Signals(4).YData = [0 1 1 1 1 1 1 1 1 0 0 0 0 0 0 0 0 0 0 0 0 0 0 0 0 0 0 0 0 0 0 0 0 0 0 0 0 0 0 0 0 0 0 0 0 0 0 0 0 0 0 0 0 0 0 0 0 0 0 0 0 0 0 0 0 0 0 0 0 0 0 0 0 0 0 0 0 0 0 0 0 0 0 0 0 0 0 0 0 0 0 0 0 0 0 0 0 0 0 0 0]
      | sbobj.Groups(3).Signals(5).Name = 'Time'
      | sbobj.Groups(3).Signals(5).XData = [0 10 20 30 40 50 60 70 80 90 100 110 120 130 140 150 160 170 180 190 200 210 220 230 240 250 260 270 280 290 300 310 320 330 340 350 360 370 380 390 400 410 420 430 440 450 460 470 480 490 500 510 520 530 540 550 560 570 580 590 600 610 620 630 640 650 660 670 680 690 700 710 720 730 740 750 760 770 780 790 800 810 820 830 840 850 860 870 880 890 900 910 920 930 940 950 960 970 980 990 1000]
      | sbobj.Groups(3).Signals(5).YData = [0 10 20 30 40 50 60 70 80 90 100 110 120 130 140 150 160 170 180 190 200 210 220 230 240 250 260 270 280 290 300 310 320 330 340 350 360 370 380 390 400 410 420 430 440 450 460 470 480 490 500 510 520 530 540 550 560 570 580 590 600 610 620 630 640 650 660 670 680 690 700 710 720 730 740 750 760 770 780 790 800 810 820 830 840 850 860 870 880 890 900 910 920 930 940 950 960 970 980 990 1000]
      | sbobj.Groups(3).TimeRange = [0 1000]
  state_Inverter : Outport  Tag=STV Outport
  requested_State : Outport  Tag=STV Outport  Port=2
  requested_Speed : Outport  Tag=STV Outport  Port=3
  digIn : Outport  Tag=STV Outport  Port=4
  Time : Outport  Tag=STV Outport  Port=5
  wires:
  FromWs/1 -> Demux/1
  Demux/1 -> state_Inverter/1
  Demux/2 -> requested_State/1
  Demux/3 -> requested_Speed/1
  Demux/4 -> digIn/1
  Demux/5 -> Time/1

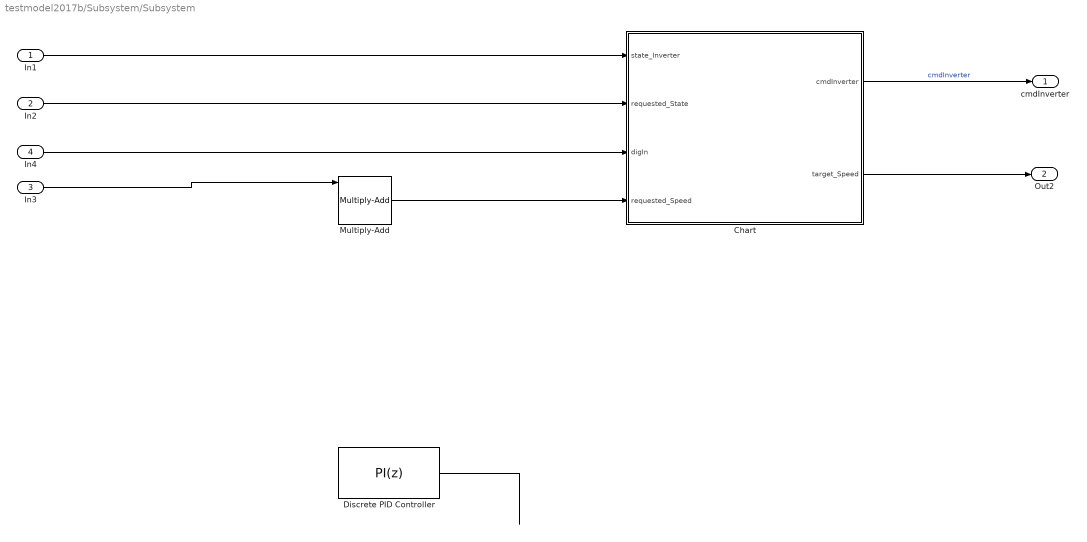
== system testmodel2017b/Subsystem/Subsystem ==
  In1 : Inport
  In2 : Inport  Port=2
  In3 : Inport  Port=3
  In4 : Inport  Port=4
  Chart : Stateflow chart  TreatAsAtomicUnit=on
  Discrete PID Controller : simulink/Continuous/PID Controller  Controller=PI  TimeDomain=Discrete-time  SampleTime=-1  IntegratorMethod=Forward Euler  FilterMethod=Forward Euler  Form=Parallel  UseFilter=on  ControllerParametersSource=internal  P=1  I=1  D=0  N=100  InitialConditionSource=external  InitialConditionForIntegrator=0  InitialConditionForFilter=0  ExternalReset=none  LimitOutput=off  UpperSaturationLimit=inf  LowerSaturationLimit=-inf  LinearizeAsGain=off  AntiWindupMode=none  Kb=1  TrackingMode=off  Kt=1  PParamMin=[]  PParamMax=[]  IParamMin=[]  IParamMax=[]  DParamMin=[]  DParamMax=[]  NParamMin=[]  NParamMax=[]  KbParamMin=[]  KbParamMax=[]  KtParamMin=[]  KtParamMax=[]  POutMin=[]  POutMax=[]  IOutMin=[]  IOutMax=[]  DOutMin=[]  DOutMax=[]  NOutMin=[]  NOutMax=[]  KbOutMin=[]  KbOutMax=[]  KtOutMin=[]  KtOutMax=[]  IntegratorOutMin=[]  IntegratorOutMax=[]  FilterOutMin=[]  FilterOutMax=[]  SumOutMin=[]  SumOutMax=[]  SumI1OutMin=[]  SumI1OutMax=[]  SumI2OutMin=[]  SumI2OutMax=[]  SumI3OutMin=[]  SumI3OutMax=[]  SumDOutMin=[]  SumDOutMax=[]  SaturationOutMin=[]  SaturationOutMax=[]  IntegratorContinuousStateAttributes=''  IntegratorStateMustResolveToSignalObject=off  IntegratorRTWStateStorageClass=Auto  FilterContinuousStateAttributes=''  FilterStateMustResolveToSignalObject=off  FilterRTWStateStorageClass=Auto  DifferentiatorICPrevScaledInput=0  DifferentiatorOutMin=[]  DifferentiatorOutMax=[]  InitialConditionSetting=State (most efficient)  FilterDiffOutCoefMin=[]  FilterDiffOutCoefMax=[]  SumDenOutMin=[]  SumDenOutMax=[]  SumNumOutMin=[]  SumNumOutMax=[]  ReciprocalOutMin=[]  ReciprocalOutMax=[]  DivideOutMin=[]  DivideOutMax=[]  TunerSelectOption=Transfer Function Based (PID Tuner App)
  Multiply-Add : hdlsllib/HDL Operations/Multiply-Add  Function=c-(a.*b)  datatype=Inherit: Inherit via internal rule  DoSatur=off
      settings: SourceProductName=HDL Coder  SourceProductBaseCode=HD
  cmdInverter : Outport
  Out2 : Outport  Port=2
  wires:
  Chart/1(cmdInverter) -> cmdInverter/1  "cmdInverter"
  Chart/2(target_Speed) -> Out2/1
  In3/1 -> Multiply-Add/1
  In2/1 -> Chart/2(requested_State)
  In4/1 -> Chart/3(digIn)
  In1/1 -> Chart/1(state_Inverter)
  Discrete PID Controller/1 -> ?
  Multiply-Add/1 -> Chart/4(requested_Speed)

== matlab function testmodel2017b/Subsystem/Truth Table ==
  data: state_Inverter input uint8; cmd output double; target_Speed output double; inSpeed input uint16
function [cmd, target_Speed] = fcn(state_Inverter, inSpeed)

aVarTruthTableCondition_1 = false;
aVarTruthTableCondition_2 = false;
aVarTruthTableCondition_3 = false;
aVarTruthTableCondition_4 = false;
aVarTruthTableCondition_5 = false;


% Example condition 1

aVarTruthTableCondition_1 = logical(state_Inverter == 0);

% Example condition 2

aVarTruthTableCondition_2 = logical(state_Inverter == 1);


aVarTruthTableCondition_3 = logical(state_Inverter == 2);


aVarTruthTableCondition_4 = logical(state_Inverter == 3);


aVarTruthTableCondition_5 = logical(state_Inverter == 4);

if (aVarTruthTableCondition_1 && ~aVarTruthTableCondition_2 && ~aVarTruthTableCondition_3 && ~aVarTruthTableCondition_4 && ~aVarTruthTableCondition_5)
    aFcnTruthTableAction_1();
elseif (aVarTruthTableCondition_1 && aVarTruthTableCondition_2 && ~aVarTruthTableCondition_3 && ~aVarTruthTableCondition_4 && ~aVarTruthTableCondition_5)
    aFcnTruthTableAction_2();
elseif (aVarTruthTableCondition_1 && aVarTruthTableCondition_2 && aVarTruthTableCondition_3 && aVarTruthTableCondition_4 && ~aVarTruthTableCondition_5)
    aFcnTruthTableAction_3();
elseif (aVarTruthTableCondition_1 && aVarTruthTableCondition_2 && aVarTruthTableCondition_3 && aVarTruthTableCondition_4 && aVarTruthTableCondition_5)
    aFcnTruthTableAction_3();
else % Default
    aFcnTruthTableAction_3();
end

function aFcnTruthTableAction_1()

% Example action 1 called from D1 & D2 column in condition table

cmd = 0
target_Speed = 0

function aFcnTruthTableAction_2()

% Example action 2 called from D3 column in condition table

cmd = 0
target_Speed = 0

function aFcnTruthTableAction_3()


cmd = 0
target_Speed = 0

== stateflow chart testmodel2017b/Subsystem/Subsystem/Chart ==
  state STOP
    du:target_Speed = 0;
  state GOTO_OPERATIONAL
    du:cmdInverter = CMD_INVERTER_GOTO_OPERATIONAL
  state OPERATIONAL
    du:target_Speed = 0;
  state GOTO_READY
    du:cmdInverter = CMD_INVERTER_GOTO_READY
  state GOTO_RUN
    du:cmdInverter = CMD_INVERTER_RUN_FWD
  state READY
    du:target_Speed = 0;
  state RUN
    du:target_Speed = requested_Speed;
  (default) -> STOP
  STOP -> GOTO_OPERATIONAL [order 1] : [requested_State == INVERTER_OPERATIONAL &&...
      | requested_State != state_Inverter]
  GOTO_OPERATIONAL -> STOP : [requested_State == state_Inverter]
  STOP -> OPERATIONAL [order 2] : [state_Inverter  >= INVERTER_OPERATIONAL]
  OPERATIONAL -> STOP [order 1] : [state_Inverter  < INVERTER_CONNECTED]
  OPERATIONAL -> GOTO_READY [order 2] : [requested_State == INVERTER_READY &&...
      | requested_State != state_Inverter &&...
      | digIn == true]
  GOTO_READY -> OPERATIONAL : [requested_State == state_Inverter]
  OPERATIONAL -> READY [order 3] : [state_Inverter  >= INVERTER_READY &&...
      | digIn == true]
  READY -> OPERATIONAL [order 1] : [state_Inverter  < INVERTER_READY]
  READY -> GOTO_RUN [order 2] : [requested_State == INVERTER_RUN_FWD &&...
      | requested_State != state_Inverter &&...
      | digIn == true]
  GOTO_RUN -> READY : [requested_State == state_Inverter]
  READY -> RUN [order 3] : [state_Inverter  >= INVERTER_RUN_FWD &&...
      | digIn == true]
  RUN -> READY : [state_Inverter  < INVERTER_RUN_FWD]
  data: state_Inverter input; requested_State input; INVERTER_STOP parameter; INVERTER_CONNECTED parameter; INVERTER_RUN_FWD parameter; INVERTER_READY parameter; CMD_INVERTER_GOTO_OPERATIONAL parameter; INVERTER_OPERATIONAL parameter; cmdInverter output double; target_Speed output double; CMD_INVERTER_GOTO_READY parameter; CMD_INVERTER_RUN_FWD parameter; digIn input; requested_Speed input

== stateflow chart testmodel2017b/Subsystem/State Transition Table ==
  state STOP
    state GOTO_OPERATIONAL
    (default) -> GOTO_OPERATIONAL
    GOTO_OPERATIONAL -> (junction 130) : [requested_State  >=INVERTER_CONNECTED]
        | {cmdInverter = CMD_INVERTER_GOTO_OPERATIONAL}
    (junction 130) -> GOTO_OPERATIONAL
  state OPERATIONAL
    state GOTO_READY
    (default) -> GOTO_READY
    GOTO_READY -> (junction 153) : [requested_State  >=INVERTER_READY]
        | {cmdInverter = CMD_INVERTER_GOTO_READY}
    (junction 153) -> GOTO_READY
  state READY
  state RUN
  (default) -> STOP
  STOP -> (junction 123) [order 2] : [requested_State  < INVERTER_CONNECTED ]
      | {cmdInverter = CMD_INVERTER_GOTO_STOP}
  (junction 123) -> STOP
  STOP -> OPERATIONAL [order 1] : [state_Inverter  >= INVERTER_CONNECTED]
  OPERATIONAL -> STOP [order 3] : [requested_State  < INVERTER_READY ]
      | {cmdInverter = CMD_INVERTER_GOTO_OPERATIONAL}
  OPERATIONAL -> (junction 105) [order 2] : [requested_State  >= INVERTER_CONNECTED]
      | {cmdInverter = CMD_INVERTER_GOTO_READY}
  (junction 105) -> OPERATIONAL
  OPERATIONAL -> READY [order 1] : [state_Inverter  >= INVERTER_READY ]
  READY -> OPERATIONAL [order 3] : [requested_State  < INVERTER_RUN_FWD ]
      | {cmdInverter = CMD_INVERTER_GOTO_OPERATIONAL}
  READY -> (junction 108) [order 2] : [requested_State  == INVERTER_RUN_FWD ]
      | {cmdInverter = CMD_INVERTER_RUN_FWD}
  (junction 108) -> READY
  READY -> RUN [order 1] : [state_Inverter  >= INVERTER_RUN_FWD & requested_Speed >= 0]
  RUN -> READY [order 2] : [requested_Speed == 0]
      | {cmdInverter = CMD_INVERTER_GOTO_READY}
  RUN -> (junction 49) [order 1] : [requested_Speed > 0]
      | {target_Speed = requested_Speed}
  (junction 49) -> RUN
  data: state_Inverter input uint8; INVERTER_CONNECTED parameter; INVERTER_READY parameter; INVERTER_RUN_FWD parameter; requested_Speed input uint16; requested_State input uint8; cmdInverter output uint8; target_Speed output uint16; CMD_INVERTER_RUN_FWD parameter; INVERTER_STOP parameter; CMD_INVERTER_GOTO_READY parameter; CMD_INVERTER_GOTO_OPERATIONAL parameter; CMD_INVERTER_GOTO_STOP parameter
